simulink model "Falling_SRA_Mathematica_Derived"  (R2022a)
settings: Solver=ode15s  StartTime=0.0  StopTime=10.0  MaxStep=0.00001  MinStep=0.0000000001  RelTol=1e-5
settings Model: Creator=yalun  LastModifiedBy=yalun
settings SolverCC: InitialStep=0.0000000001
settings RTWCC: GenCodeOnly=on

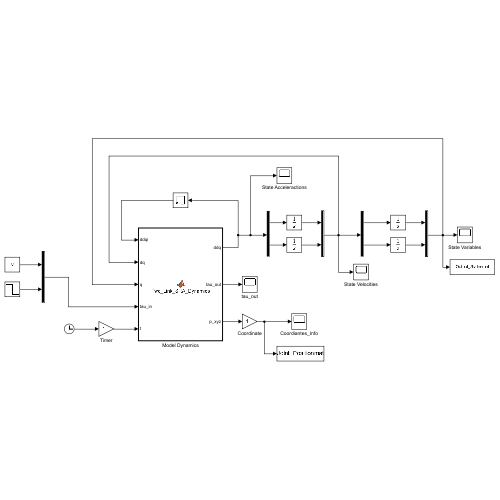
[thumbnail: Simulink's stored preview of the top-level diagram]
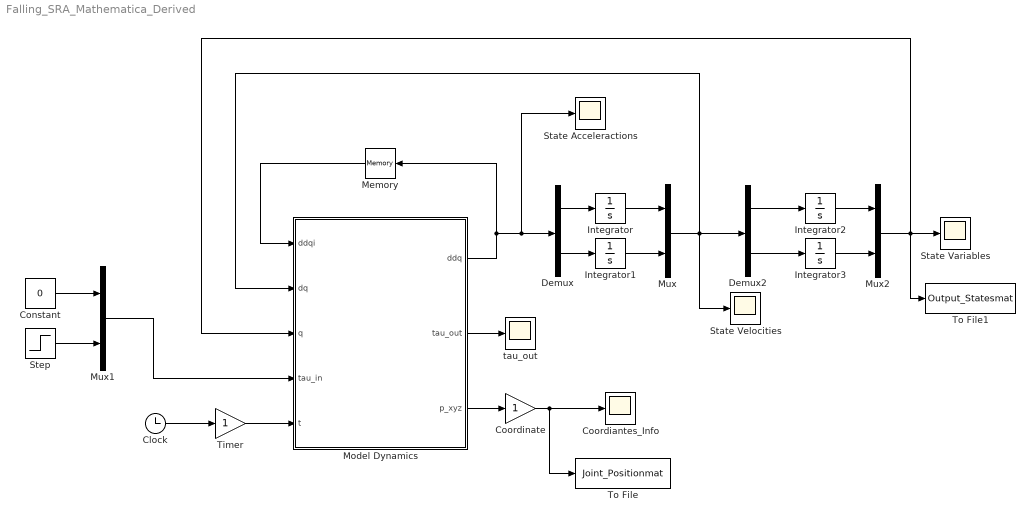
== system Falling_SRA_Mathematica_Derived ==
  Clock : Clock
  Constant : Constant  Value=0
  Coordiantes_Info : Scope
  Coordinate : Gain
  Demux : Demux  Outputs=2
  Demux2 : Demux  Outputs=2
  Integrator{,1..3} (4 alike) : Integrator
  Memory : Memory
  Model Dynamics : MATLAB Function  TreatAsAtomicUnit=on
      settings: ErrorFcn=StateflowTranslatetranslate
  Mux : Mux  Inputs=2
  Mux1 : Mux  Inputs=2
  Mux2 : Mux  Inputs=2
  State Acceleractions : Scope
  State Variables : Scope
  State Velocities : Scope
  Step : Step  Before=003  After=0  SampleTime=0
  Timer : Gain
  To File : ToFile  Filename=Joint_Positionmat  SaveFormat=Timeseries
  To File1 : ToFile  Filename=Output_Statesmat  SaveFormat=Timeseries
  tau_out : Scope
  wires:
  Timer/1 -> Model Dynamics/5(t)
  Clock/1 -> Timer/1
  Model Dynamics/1(ddq) -> State Acceleractions/1, Demux/1, Memory/1
  Memory/1 -> Model Dynamics/1(ddqi)
  Model Dynamics/2(tau_out) -> tau_out/1
  Model Dynamics/3(p_xyz) -> Coordinate/1
  Coordinate/1 -> To File/1, Coordiantes_Info/1
  Integrator/1 -> Mux/1
  Integrator1/1 -> Mux/2
  Demux/1 -> Integrator/1
  Demux/2 -> Integrator1/1
  Mux/1 -> State Velocities/1, Model Dynamics/2(dq), Demux2/1
  Demux2/1 -> Integrator2/1
  Integrator3/1 -> Mux2/2
  Demux2/2 -> Integrator3/1
  Integrator2/1 -> Mux2/1
  Mux2/1 -> To File1/1, Model Dynamics/3(q), State Variables/1
  Mux1/1 -> Model Dynamics/4(tau_in)
  Constant/1 -> Mux1/1
  Step/1 -> Mux1/2

== matlab function Falling_SRA_Mathematica_Derived/Model Dynamics ==
  data: ddqi input size=2; ddq output size=2; tau_out output size=2; dq input size=2; q input size=2; tau_in input size=2; t input size=1; p_xyz output size=4
function [ddq,tau_out,p_xyz] = Two_Link_SRA_Dynamics(ddqi,dq,q,tau_in,t)

% Similar to C or C++, we have to claim the function we are going to use
% externally
coder.extrinsic('sym');
coder.extrinsic('symfun');
coder.extrinsic('jacobian');
coder.extrinsic('diff');
coder.extrinsic('subs');
coder.extrinsic('double');

% Fixed position in inertia frame
pfx=-1;
pfy=1;

% The number of link for each side of the SRA
n_link=2;
ddq=zeros(n_link,1);
tau_out=zeros(n_link,1);

%% SRA Parameters %%
% Segment stiffness
k=[2.5,2];
% Segment damping coefficient
b=[1,0.9];
% Segment length & mass
L=[0.3,0.3];
m=[1.25,1.25];

g=9.81;
M=zeros(n_link,n_link);
C=zeros(n_link,n_link);
%% End %%

theta1=q(1);
theta2=q(2);

theta1dot=dq(1);
theta2dot=dq(2);

m1=m(1);
m2=m(2);
L1=L(1);
L2=L(2);



% M=[(1/48).*L1.^2.*m1+(1/48).*L2.^2.*m2+L1.^2.*m1.*theta1.^(-4).*...
%   (2+theta1.^2+(-2).*cos(theta1)+(-2).*theta1.*sin(theta1))...
% +m2.*theta1.^(-4).*theta2.^(-2).*((theta1.*(L2.*theta1+(-1).*L1.*theta2).*cos(theta1)+(-1).*L2.*theta1.^2.* ...
%   cos(theta1+theta2)+L1.*theta2.*sin(theta1)).^2+(L1.*theta2+(-1).*L1.*theta2.*cos(theta1) ...
%   +theta1.*(L2.*theta1+(-1).*L1.*theta2).*sin(theta1)+(-1)...
% .*L2.*theta1.^2.*sin(theta1+ ...
%   theta2)).^2),(1/48).*L2.*m2.*theta1.^(-2).*theta2.^(-2).*((-48).*L1+48.*L2.*theta1.^2+L2.*theta1.^2.*theta2.^2+48.*L1.*cos(theta1)+48.*(L1+(-1).* ...
%   L2.*theta1.^2+L1.*theta1.*theta2).*cos(theta2)+(-48).*L1.*cos(theta1+theta2)+(-48).* ...
%   L1.*theta1.*sin(theta2)+48.*L1.*theta2.*sin(theta2)+(-48).*L1.*theta2.*sin(theta1+ ...
%   theta2));(1/48).*L2.*m2.*theta1.^(-2).*theta2.^(-2).*((-48).*L1+48.*L2.* ...
%   theta1.^2+L2.*theta1.^2.*theta2.^2+48.*L1.*cos(theta1)+...
% 48.*(L1+(-1).*L2.* ...
%   theta1.^2+L1.*theta1.*theta2).*cos(theta2)+(-48).*L1.*...
% cos(theta1+theta2)+(-48).*L1.* ...
%   theta1.*sin(theta2)+48.*L1.*theta2.*sin(theta2)+(-48).*...
% L1.*theta2.*sin(theta1+theta2)),( ...
%   1/48).*L2.^2.*m2.*theta2.^(-4).*(96+48.*theta2.^2+theta2.^...
% 4+(-96).*cos(theta2)+(-96).*theta2.*sin(theta2))];

% 2022.10.31
% The 4 by 4 matrix cannot be successfully derived in Simulink for the
% whole matrix, only the single element can be expressed, the reason behind
% should be analyzed afterwards.

M(1,1)=(1/48).*L1.^2.*m1+(1/48).*L2.^2.*m2+L1.^2.*m1.*theta1.^(-4).*(2+theta1.^2+(-2).*cos(theta1)+(-2).*theta1.*sin(theta1))+m2.*theta1.^(-4).*theta2.^(-2).*((theta1.*(L2.*theta1+(-1).*L1.*theta2).*cos(theta1)+(-1).*L2.*theta1.^2.* ...
  cos(theta1+theta2)+L1.*theta2.*sin(theta1)).^2+(L1.*theta2+(-1).*L1.*theta2.*cos(theta1) ...
  +theta1.*(L2.*theta1+(-1).*L1.*theta2).*sin(theta1)+(-1)...
.*L2.*theta1.^2.*sin(theta1+ ...
  theta2)).^2);
M(1,2)=(1/48).*L2.*m2.*theta1.^(-2).*theta2.^(-2).*((-48).*L1+48.*L2.*theta1.^2+L2.*theta1.^2.*theta2.^2+48.*L1.*cos(theta1)+48.*(L1+(-1).* ...
  L2.*theta1.^2+L1.*theta1.*theta2).*cos(theta2)+(-48).*L1.*cos(theta1+theta2)+(-48).* ...
  L1.*theta1.*sin(theta2)+48.*L1.*theta2.*sin(theta2)+(-48).*L1.*theta2.*sin(theta1+ ...
  theta2));
M(2,1)=(1/48).*L2.*m2.*theta1.^(-2).*theta2.^(-2).*((-48).*L1+48.*L2.* ...
  theta1.^2+L2.*theta1.^2.*theta2.^2+48.*L1.*cos(theta1)+...
48.*(L1+(-1).*L2.* ...
  theta1.^2+L1.*theta1.*theta2).*cos(theta2)+(-48).*L1.*...
cos(theta1+theta2)+(-48).*L1.* ...
  theta1.*sin(theta2)+48.*L1.*theta2.*sin(theta2)+(-48).*...
L1.*theta2.*sin(theta1+theta2));
M(2,2)=(1/48).*L2.^2.*m2.*theta2.^(-4).*(96+48.*theta2.^2+theta2.^...
4+(-96).*cos(theta2)+(-96).*theta2.*sin(theta2));



C=[(1/2).*theta1dot.*(L1.^2.*m1.*theta1.^(-4).*(2.*theta1+(-2).*theta1.*cos( ...
  theta1))+(-4).*L1.^2.*m1.*theta1.^(-5).*(2+theta1.^2+(-2).*cos(theta1)+(-2) ...
  .*theta1.*sin(theta1))+(-4).*m2.*theta1.^(-5).*theta2.^(-2).*((theta1.*(L2.*theta1+( ...
  -1).*L1.*theta2).*cos(theta1)+(-1).*L2.*theta1.^2.*cos(theta1+theta2)+L1.*theta2.* ...
  sin(theta1)).^2+(L1.*theta2+(-1).*L1.*theta2.*cos(theta1)+theta1.*(L2.*theta1+(-1).* ...
  L1.*theta2).*sin(theta1)+(-1).*L2.*theta1.^2.*sin(theta1+theta2)).^2)+m2.*theta1.^( ...
  -4).*theta2.^(-2).*(2.*(theta1.*(L2.*theta1+(-1).*L1.*theta2).*cos(theta1)+(-1) ...
  .*L2.*theta1.^2.*cos(theta1+theta2)+L2.*theta1.*sin(theta1)+L1.*theta2.*sin(theta1)+( ...
  L2.*theta1+(-1).*L1.*theta2).*sin(theta1)+(-2).*L2.*theta1.*sin(theta1+theta2)).*( ...
  L1.*theta2+(-1).*L1.*theta2.*cos(theta1)+theta1.*(L2.*theta1+(-1).*L1.*theta2).*sin( ...
  theta1)+(-1).*L2.*theta1.^2.*sin(theta1+theta2))+2.*(theta1.*(L2.*theta1+(-1).*L1.* ...
  theta2).*cos(theta1)+(-1).*L2.*theta1.^2.*cos(theta1+theta2)+L1.*theta2.*sin(theta1)).*( ...
  L2.*theta1.*cos(theta1)+L1.*theta2.*cos(theta1)+(L2.*theta1+(-1).*L1.*theta2).*cos( ...
  theta1)+(-2).*L2.*theta1.*cos(theta1+theta2)+(-1).*theta1.*(L2.*theta1+(-1).*L1.*theta2) ...
  .*sin(theta1)+L2.*theta1.^2.*sin(theta1+theta2))))+(1/2).*theta2dot.*(L1.^2.* ...
  m1.*theta1.^(-4).*(2.*theta1+(-2).*theta1.*cos(theta1))+(-4).*L1.^2.*m1.* ...
  theta1.^(-5).*(2+theta1.^2+(-2).*cos(theta1)+(-2).*theta1.*sin(theta1))+(-1/48) ...
  .*L2.*m2.*theta1.^(-2).*theta2.^(-2).*(96.*L2.*theta1+2.*L2.*theta1.*theta2.^2+ ...
  48.*((-2).*L2.*theta1+L1.*theta2).*cos(theta2)+(-48).*L1.*theta2.*cos(theta1+theta2) ...
  +(-48).*L1.*sin(theta1)+(-48).*L1.*sin(theta2)+48.*L1.*sin(theta1+theta2))+( ...
  1/24).*L2.*m2.*theta1.^(-3).*theta2.^(-2).*((-48).*L1+48.*L2.*theta1.^2+ ...
  L2.*theta1.^2.*theta2.^2+48.*L1.*cos(theta1)+48.*(L1+(-1).*L2.*theta1.^2+ ...
  L1.*theta1.*theta2).*cos(theta2)+(-48).*L1.*cos(theta1+theta2)+(-48).*L1.*theta1.* ...
  sin(theta2)+48.*L1.*theta2.*sin(theta2)+(-48).*L1.*theta2.*sin(theta1+theta2))+(-2) ...
  .*m2.*theta1.^(-4).*theta2.^(-3).*((theta1.*(L2.*theta1+(-1).*L1.*theta2).*cos( ...
  theta1)+(-1).*L2.*theta1.^2.*cos(theta1+theta2)+L1.*theta2.*sin(theta1)).^2+(L1.*theta2+ ...
  (-1).*L1.*theta2.*cos(theta1)+theta1.*(L2.*theta1+(-1).*L1.*theta2).*sin(theta1)+( ...
  -1).*L2.*theta1.^2.*sin(theta1+theta2)).^2)+(-4).*m2.*theta1.^(-5).*theta2.^(-2) ...
  .*((theta1.*(L2.*theta1+(-1).*L1.*theta2).*cos(theta1)+(-1).*L2.*theta1.^2.*cos( ...
  theta1+theta2)+L1.*theta2.*sin(theta1)).^2+(L1.*theta2+(-1).*L1.*theta2.*cos(theta1)+ ...
  theta1.*(L2.*theta1+(-1).*L1.*theta2).*sin(theta1)+(-1).*L2.*theta1.^2.*sin(theta1+ ...
  theta2)).^2)+m2.*theta1.^(-4).*theta2.^(-2).*(2.*(L1+(-1).*L1.*cos(theta1)+( ...
  -1).*L2.*theta1.^2.*cos(theta1+theta2)+(-1).*L1.*theta1.*sin(theta1)).*(L1.*theta2+( ...
  -1).*L1.*theta2.*cos(theta1)+theta1.*(L2.*theta1+(-1).*L1.*theta2).*sin(theta1)+(-1) ...
  .*L2.*theta1.^2.*sin(theta1+theta2))+2.*(theta1.*(L2.*theta1+(-1).*L1.*theta2).*cos( ...
  theta1)+(-1).*L2.*theta1.^2.*cos(theta1+theta2)+L1.*theta2.*sin(theta1)).*((-1).* ...
  L1.*theta1.*cos(theta1)+L1.*sin(theta1)+L2.*theta1.^2.*sin(theta1+theta2)))+m2.* ...
  theta1.^(-4).*theta2.^(-2).*(2.*(theta1.*(L2.*theta1+(-1).*L1.*theta2).*cos(theta1)+ ...
  (-1).*L2.*theta1.^2.*cos(theta1+theta2)+L2.*theta1.*sin(theta1)+L1.*theta2.*sin(theta1)+ ...
  (L2.*theta1+(-1).*L1.*theta2).*sin(theta1)+(-2).*L2.*theta1.*sin(theta1+theta2)).*( ...
  L1.*theta2+(-1).*L1.*theta2.*cos(theta1)+theta1.*(L2.*theta1+(-1).*L1.*theta2).*sin( ...
  theta1)+(-1).*L2.*theta1.^2.*sin(theta1+theta2))+2.*(theta1.*(L2.*theta1+(-1).*L1.* ...
  theta2).*cos(theta1)+(-1).*L2.*theta1.^2.*cos(theta1+theta2)+L1.*theta2.*sin(theta1)).*( ...
  L2.*theta1.*cos(theta1)+L1.*theta2.*cos(theta1)+(L2.*theta1+(-1).*L1.*theta2).*cos( ...
  theta1)+(-2).*L2.*theta1.*cos(theta1+theta2)+(-1).*theta1.*(L2.*theta1+(-1).*L1.*theta2) ...
  .*sin(theta1)+L2.*theta1.^2.*sin(theta1+theta2)))),(1/2).*theta2dot.*((1/24).* ...
  L2.*m2.*theta1.^(-2).*theta2.^(-2).*(2.*L2.*theta1.^2.*theta2+48.*L1.*theta2.* ...
  cos(theta2)+(-48).*L1.*theta2.*cos(theta1+theta2)+48.*L1.*sin(theta2)+(-48).*( ...
  L1+(-1).*L2.*theta1.^2+L1.*theta1.*theta2).*sin(theta2))+(-1/12).*L2.*m2.* ...
  theta1.^(-2).*theta2.^(-3).*((-48).*L1+48.*L2.*theta1.^2+L2.*theta1.^2.* ...
  theta2.^2+48.*L1.*cos(theta1)+48.*(L1+(-1).*L2.*theta1.^2+L1.*theta1.*theta2).* ...
  cos(theta2)+(-48).*L1.*cos(theta1+theta2)+(-48).*L1.*theta1.*sin(theta2)+48.* ...
  L1.*theta2.*sin(theta2)+(-48).*L1.*theta2.*sin(theta1+theta2)))+(1/2).*theta1dot.*(( ...
  -2).*m2.*theta1.^(-4).*theta2.^(-3).*((theta1.*(L2.*theta1+(-1).*L1.*theta2).* ...
  cos(theta1)+(-1).*L2.*theta1.^2.*cos(theta1+theta2)+L1.*theta2.*sin(theta1)).^2+( ...
  L1.*theta2+(-1).*L1.*theta2.*cos(theta1)+theta1.*(L2.*theta1+(-1).*L1.*theta2).*sin( ...
  theta1)+(-1).*L2.*theta1.^2.*sin(theta1+theta2)).^2)+m2.*theta1.^(-4).*theta2.^(-2) ...
  .*(2.*(L1+(-1).*L1.*cos(theta1)+(-1).*L2.*theta1.^2.*cos(theta1+theta2)+(-1) ...
  .*L1.*theta1.*sin(theta1)).*(L1.*theta2+(-1).*L1.*theta2.*cos(theta1)+theta1.*(L2.* ...
  theta1+(-1).*L1.*theta2).*sin(theta1)+(-1).*L2.*theta1.^2.*sin(theta1+theta2))+2.*( ...
  theta1.*(L2.*theta1+(-1).*L1.*theta2).*cos(theta1)+(-1).*L2.*theta1.^2.*cos(theta1+ ...
  theta2)+L1.*theta2.*sin(theta1)).*((-1).*L1.*theta1.*cos(theta1)+L1.*sin(theta1)+ ...
  L2.*theta1.^2.*sin(theta1+theta2))));(1/2).*theta1dot.*((1/24).*L2.*m2.* ...
  theta1.^(-2).*theta2.^(-2).*(96.*L2.*theta1+2.*L2.*theta1.*theta2.^2+48.*((-2).* ...
  L2.*theta1+L1.*theta2).*cos(theta2)+(-48).*L1.*theta2.*cos(theta1+theta2)+(-48).* ...
  L1.*sin(theta1)+(-48).*L1.*sin(theta2)+48.*L1.*sin(theta1+theta2))+(-1/12).* ...
  L2.*m2.*theta1.^(-3).*theta2.^(-2).*((-48).*L1+48.*L2.*theta1.^2+L2.* ...
  theta1.^2.*theta2.^2+48.*L1.*cos(theta1)+48.*(L1+(-1).*L2.*theta1.^2+L1.* ...
  theta1.*theta2).*cos(theta2)+(-48).*L1.*cos(theta1+theta2)+(-48).*L1.*theta1.*sin( ...
  theta2)+48.*L1.*theta2.*sin(theta2)+(-48).*L1.*theta2.*sin(theta1+theta2))+2.*m2.* ...
  theta1.^(-4).*theta2.^(-3).*((theta1.*(L2.*theta1+(-1).*L1.*theta2).*cos(theta1)+( ...
  -1).*L2.*theta1.^2.*cos(theta1+theta2)+L1.*theta2.*sin(theta1)).^2+(L1.*theta2+(-1) ...
  .*L1.*theta2.*cos(theta1)+theta1.*(L2.*theta1+(-1).*L1.*theta2).*sin(theta1)+(-1).* ...
  L2.*theta1.^2.*sin(theta1+theta2)).^2)+(-1).*m2.*theta1.^(-4).*theta2.^(-2).*( ...
  2.*(L1+(-1).*L1.*cos(theta1)+(-1).*L2.*theta1.^2.*cos(theta1+theta2)+(-1).* ...
  L1.*theta1.*sin(theta1)).*(L1.*theta2+(-1).*L1.*theta2.*cos(theta1)+theta1.*(L2.*theta1+ ...
  (-1).*L1.*theta2).*sin(theta1)+(-1).*L2.*theta1.^2.*sin(theta1+theta2))+2.*(theta1.* ...
  (L2.*theta1+(-1).*L1.*theta2).*cos(theta1)+(-1).*L2.*theta1.^2.*cos(theta1+theta2)+ ...
  L1.*theta2.*sin(theta1)).*((-1).*L1.*theta1.*cos(theta1)+L1.*sin(theta1)+L2.* ...
  theta1.^2.*sin(theta1+theta2)))),(1/2).*theta2dot.*((1/48).*L2.^2.*m2.*theta2.^( ...
  -4).*(96.*theta2+4.*theta2.^3+(-96).*theta2.*cos(theta2))+(-1/12).*L2.^2.* ...
  m2.*theta2.^(-5).*(96+48.*theta2.^2+theta2.^4+(-96).*cos(theta2)+(-96).*theta2.* ...
  sin(theta2)))];

Pk=[k(1)*theta1;k(2)*theta2];
Pb=[b(1)*theta1dot;b(2)*theta2dot];
Pg=[(L1*sin(theta1)/(2*theta1));
    (-L1+pfy*theta1+L1*cos(theta1))/theta1+(-L1*sin(theta1)/theta1+(L1/theta1-L2/theta2)*sin(theta1)+L2*sin(theta1+theta2)/theta2)/2];

ddq=double(M\(tau_in-C*dq-Pg-Pk-Pb));
% ddq=double(pinv(M)*(tau_in-C*dq-Pg-Pk-Pb));
tau_out=double(M*ddqi+C*dq+Pg+Pk+Pb);
p_xyz=transpose([pfx+L1*sin(theta1)/theta1,(-L1+pfy*theta1+L1*cos(theta1))/theta1,pfx+(L1/theta1-L2/theta2)*sin(theta1)+L2*sin(theta1+theta2)/theta2,(-L1*theta2+pfy*theta1*theta2+(-L2*theta1+L1*theta2)*cos(theta1)+L2*theta1*cos(theta1+theta2))/(theta1*theta2)]);

end
